simulink model "Question4part2"  (R2014b)
settings: Solver=ode45  StartTime=0.0  StopTime=10.0  FixedStep=.001  RelTol=1e-3
settings Model: Creator=zeinab  LastModifiedBy=SURENA

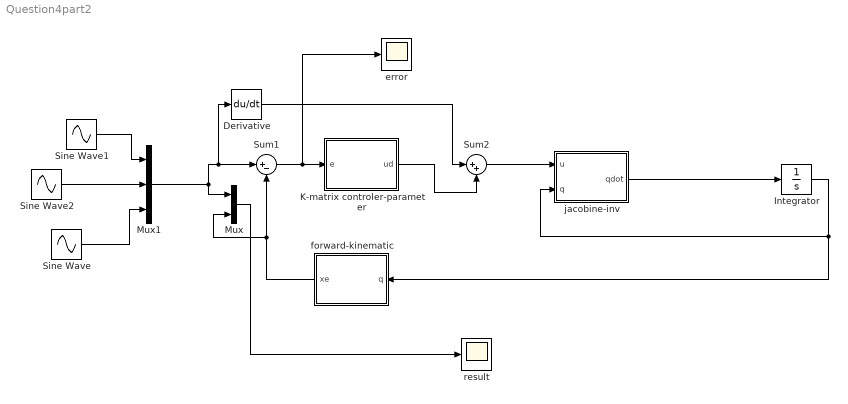
== system Question4part2 ==
  Derivative : Derivative
  Integrator : Integrator  InitialCondition=[0;.1;.2]
  K-matrix controler-parameter : MATLAB Function  TreatAsAtomicUnit=on
  Mux : Mux  Inputs=2
  Mux1 : Mux  Inputs=3
  Sine Wave : Sin  Amplitude=.2  Bias=-1  SampleTime=0
  Sine Wave1 : Sin  Amplitude=.2  Bias=1  SampleTime=0
  Sine Wave2 : Sin  Amplitude=.2  Bias=1  SampleTime=0
  Sum1 : Sum  Inputs=|+-
  Sum2 : Sum  Inputs=|++
  error : Scope
      settings: YMin=-0.014  YMax=0
  forward-kinematic : MATLAB Function  TreatAsAtomicUnit=on
  jacobine-inv : MATLAB Function  TreatAsAtomicUnit=on
  result : Scope
  wires:
  jacobine-inv/1(qdot) -> Integrator/1
  Mux1/1 -> Derivative/1, Sum1/1, Mux/1
  Integrator/1 -> forward-kinematic/1(q), jacobine-inv/2(q)
  forward-kinematic/1(xe) -> Sum1/2, Mux/2
  Sum1/1 -> error/1, K-matrix controler-parameter/1(e)
  K-matrix controler-parameter/1(ud) -> Sum2/2
  Derivative/1 -> Sum2/1
  Sum2/1 -> jacobine-inv/1(u)
  Mux/1 -> result/1
  Sine Wave/1 -> Mux1/3
  Sine Wave1/1 -> Mux1/1
  Sine Wave2/1 -> Mux1/2

== matlab function Question4part2/forward-kinematic ==
  data: xe output; q input
function xe = fcn(q)
q1 = q(1); q2 = q(2);q3 = q(3); 
xe=[cos(q1)+cos(q1+q2); sin(q1)+sin(q1+q2); -q3-1];

== matlab function Question4part2/jacobine-inv ==
  data: u input; qdot output; q input

function qdot = fcn(u,q)
q1 = q(1);q2 = q(2);
jinv=[cos(q1 + q2)/sin(q2),sin(q1 + q2)/sin(q2),0;-(cos(q1 + q2) + cos(q1))/sin(q2),-(sin(q1 + q2) + sin(q1))/sin(q2),0;0,0,-1];
qdot =  jinv * u;

== matlab function Question4part2/K-matrix controler-parameter ==
  data: ud output; e input
function ud = fcn(e)
k=eye(3);
ud = k*e;
